simulink library "EngineSystemSubmodel"  (R2014b)
settings: Solver=ode45  StartTime=0.0  StopTime=10.0  FixedStep=1e-4  RelTol=1e-3
values from neighbouring files (symbols this model uses):
  D_turb_wheel = TC.TC_map.turb.D_wheel    [init_MVM.m]
  delta = 2    [Init8RTFLEX68D.m]    (also in Untitled2.m = fcn(p); fcn.m = zeros(size(p)))
  eta_turb_max = TC.TC_map.turb.eff_max    [init_MVM.m]
  flow_coeff_turb = [-1.585326540339;-4.823836967181;1.5853156139822]    [Init8RTFLEX68D.m]    (also in init_MVM.m = TC.TC_map.turb.flow_fit_coeff)
  fs = 0.0683    [Init8RTFLEX68D.m]    (also in NOxProcessGUI.m = varargin{2}; initHybrid.m; initMV.m; init_MVM.m = 0.0682925799315)
  genset = generators(1)    [runTempCyl4S.m]
  J_tc = TC.SAE_map_comp.inertia    [init_MVM.m]
  kai = 1.7    [Init8RTFLEX68D.m]
  Kb = 1*ones(engines,1)    [initHybrid.m]    (also in initMV.m; init_MVM.m = 1; init_ele.m = 1)
  Kd = 20*ones(engines,1)    [initHybrid.m]    (also in initMV.m; init_MVM.m = 10; init_ele.m = 20)
  Ki = 20*ones(engines,1)    [initHybrid.m]    (also in initMV.m; init_MVM.m = 10; init_ele.m = 20)
  Kp = 20*ones(engines,1)    [initHybrid.m]    (also in initMV.m; init_MVM.m = 10; init_ele.m = 20)
  Load_amp = x(4) + xRef(i)    [GetErrGensetResp.m]    (also in runsimulation.m = 0.55; runsimulationRecovery.m = InitialLoad(jj) + LoadStep(ii))
  Load_bias = x(4)    [GetErrGensetResp.m]    (also in runsimulation.m = 0.15; runsimulationRecovery.m = InitialLoad(jj))
  Load_index = 1    [GetErrGensetResp.m]    (also in runsimulation.m; runsimulationRecovery.m)
  N = x*noMol    [NOxProcessGUI.m]    (also in initHybrid.m = .1*ones(engines,1); initMV.m = .1*ones(engines,1); init_ele.m = 0.1)
  omegat0 = RPM_TC_initial/30*pi    [init_MVM.m]
  Start_time = 50    [GetErrGensetResp.m]    (also in runsimulation.m; runsimulationRecovery.m)
  T_load = 1    [GetErrGensetResp.m]    (also in runsimulation.m; runsimulationRecovery.m)
  T_ref_turb = TC.TC_map.turb.T_ref    [init_MVM.m]
  u0 = 0.2    [init_MVM.m]
  Uc_opt = TC.TC_map.turb.Uc_opt    [init_MVM.m]
  uMax = 1.5*ones(engines,1)    [initHybrid.m]    (also in initMV.m; init_MVM.m = 1.1; init_ele.m = 1.1)
  uMin = 0*ones(engines,1)    [initHybrid.m]    (also in initMV.m; init_MVM.m = 0.1; init_ele.m = 0.1)
undefined symbols (not defined in the file or in its folder): CAIPO, control, CV, cyl, eng, engSCont, omega0, rhoG0, Td, Ti, turbo, u_max, volDisp, vSCont, vSDes
undefined symbols (not defined in the file): comp_eff_map, comp_flow_map, n288_rep, npr, nsp, pr_rep, vComp
libraries: EngineSystemSubmodel x167, simulink x2
(part 2 of 5)

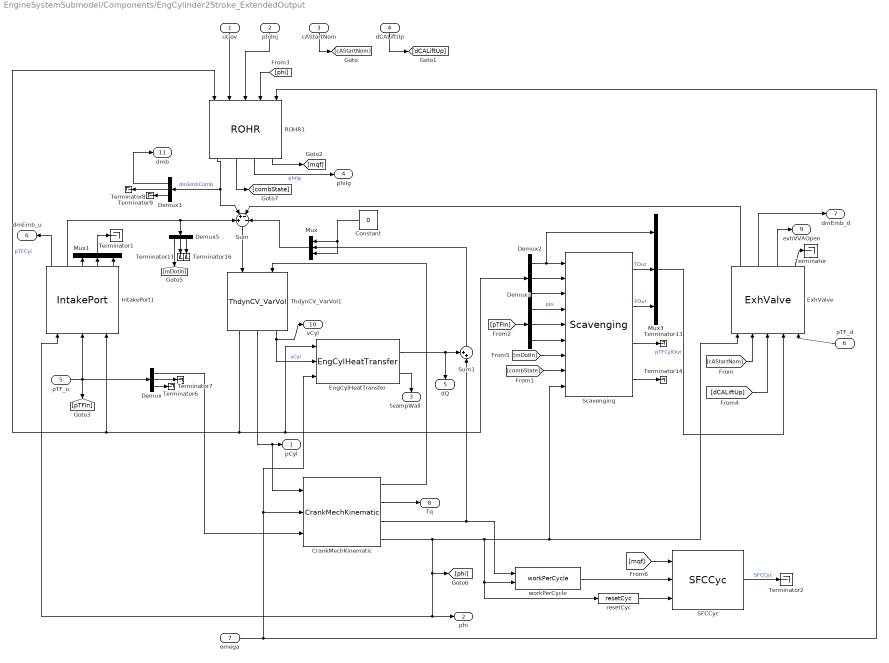
== system EngineSystemSubmodel/Components/EngCylinder2Stroke_ExtendedOutput ==
  uGov : Inport
  phiInj : Inport  Port=2
  cAStartNom : Inport  Port=3
  dCALiftUp : Inport  Port=4
  pTF_u : Inport  Port=5
  pTF_d : Inport  Port=6
  omega : Inport  Port=7
  Constant : Constant  Value=0
  CrankMechKinematic : EngineSystemSubmodel/Mechanical Part/CrankMechKinematic
  Demux{,1..3,5} (5 alike) : Demux  Outputs=3
  EngCylHeatTransfer : EngineSystemSubmodel/Heat Transfer/EngCylHeatTransfer
  ExhValve : EngineSystemSubmodel/Components/ExhValve
  IntakePort1 : EngineSystemSubmodel/Components/IntakePort
  Mux : Mux  Inputs=3
  Mux1 : Mux  Inputs=3
  Mux3 : Mux  Inputs=3
  ROHR1 : EngineSystemSubmodel/Combustion/ROHR
  SFCCyc : EngineSystemSubmodel/EngineOperatingParameterCalculation/SFCCyc
  Scavenging : EngineSystemSubmodel/Gas Exchange/Scavenging
  Sum : Sum  Inputs=++--
  Sum1 : Sum  Inputs=++|
  Terminator{,1..2,6..9,11,13..14,16} (11 alike) : Terminator
  ThdynCV_VarVol1 : EngineSystemSubmodel/Control Volume/ThdynCV_VarVol  CV=cyl.init
  resetCyc : EngineSystemSubmodel/EngineOperatingParameterCalculation/resetCyc
  workPerCycle : EngineSystemSubmodel/EngineOperatingParameterCalculation/workPerCycle
  pCyl : Outport
  phi : Outport  Port=2
  teampWall : Outport  Port=3
  phiIg : Outport  Port=4
  dQ : Outport  Port=5
  dmEmb_u : Outport  Port=6
  dmEmb_d : Outport  Port=7
  Tq : Outport  Port=8
  exhVVAOpen : Outport  Port=9
  vCyl : Outport  Port=10
  dmb : Outport  Port=11
  wires:
  SFCCyc/1 -> Terminator2/1  "SFCCyc"
  [mqf] -> SFCCyc/1
  workPerCycle/1 -> SFCCyc/2
  resetCyc/1 -> SFCCyc/3
  Mux3/1 -> ExhValve/4  "pTFCylOut"
  [cAStartNom] -> ExhValve/2
  dCALiftUp/1 -> [dCALiftUp]
  cAStartNom/1 -> [cAStartNom]
  ExhValve/2 -> dmEmb_d/1
  ExhValve/4 -> Terminator/1
  ExhValve/3 -> exhVVAOpen/1
  Mux1/1 -> Terminator1/1
  IntakePort1/5 -> Mux1/3
  IntakePort1/4 -> Mux1/2
  IntakePort1/3 -> Mux1/1
  ROHR1/3 -> phiIg/1  "phiIg"
  EngCylHeatTransfer/2 -> teampWall/1
  Demux/3 -> Terminator7/1
  Demux/2 -> Terminator6/1
  Constant/1 -> Mux/3, Mux/1
  Mux/1 -> Sum/4
  Sum1/1 -> Mux/2
  EngCylHeatTransfer/1 -> Sum1/1, dQ/1
  ThdynCV_VarVol1/3 -> EngCylHeatTransfer/2, vCyl/1  "vCyl"
  IntakePort1/1 -> dmEmb_u/1
  omega/1 -> ROHR1/5, EngCylHeatTransfer/3, CrankMechKinematic/2
  phiInj/1 -> ROHR1/3
  CrankMechKinematic/2 -> Tq/1
  Demux/1 -> CrankMechKinematic/3
  CrankMechKinematic/3 -> Sum1/2, workPerCycle/1
  uGov/1 -> ROHR1/2
  CrankMechKinematic/1 -> ThdynCV_VarVol1/2
  ThdynCV_VarVol1/2 -> CrankMechKinematic/1, pCyl/1
  ThdynCV_VarVol1/1 -> EngCylHeatTransfer/1, Demux2/1, IntakePort1/3, ROHR1/1  "pTFCyl"
  Sum/1 -> ThdynCV_VarVol1/1
  ExhValve/1 -> Sum/3
  ROHR1/1 -> Sum/2, Demux1/1  "dmEmbComb"
  Demux1/1 -> dmb/1
  Demux1/2 -> Terminator8/1
  Demux1/3 -> Terminator9/1
  ROHR1/4 -> [mqf]
  pTF_u/1 -> [pTFIn], Demux/1, IntakePort1/2
  pTF_d/1 -> ExhValve/5
  ROHR1/2 -> [combState]
  [pTFIn] -> Demux3/1
  Demux3/1 -> Scavenging/4  "pIn"
  Demux3/2 -> Scavenging/5
  Demux3/3 -> Scavenging/6
  [mDotIn] -> Scavenging/7
  CrankMechKinematic/4 -> [phi], IntakePort1/1, phi/1, Scavenging/9, ExhValve/1, workPerCycle/2, resetCyc/1
  IntakePort1/2 -> Demux5/1, Sum/1
  Demux5/2 -> Terminator11/1
  Demux5/3 -> Terminator16/1
  Demux5/1 -> [mDotIn]
  [combState] -> Scavenging/8
  [phi] -> ROHR1/4
  Scavenging/3 -> Terminator13/1
  Scavenging/4 -> Terminator14/1
  Demux2/2 -> Scavenging/2
  Demux2/1 -> Mux3/1, Scavenging/1
  Demux2/3 -> Scavenging/3
  Scavenging/1 -> Mux3/2  "TOut"
  Scavenging/2 -> Mux3/3  "FOut"
  [dCALiftUp] -> ExhValve/3

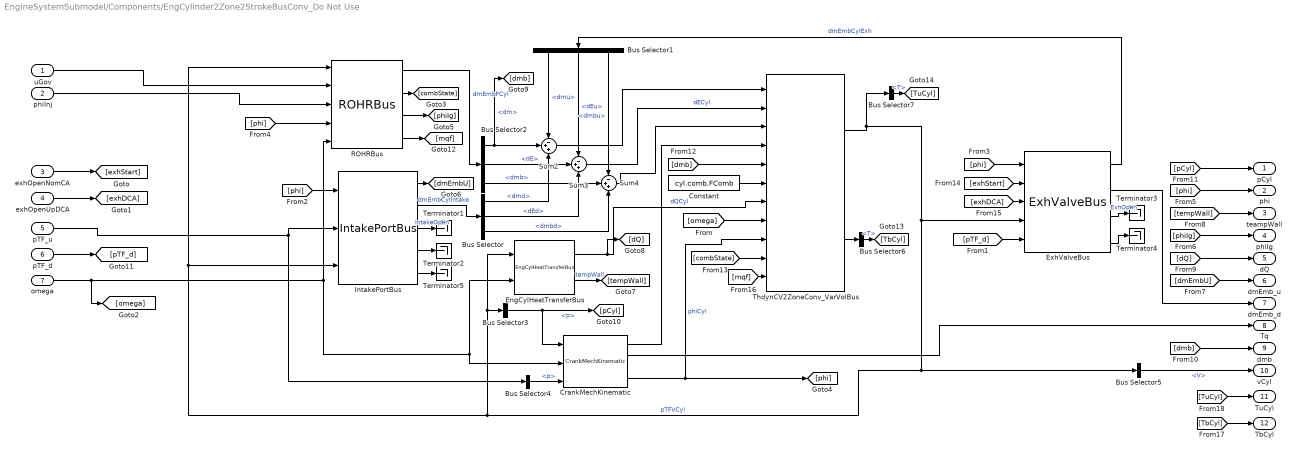
== system EngineSystemSubmodel/Components/EngCylinder2Zone2StrokeBusConv_Do Not Use ==
  uGov : Inport
  phiInj : Inport  Port=2
  exhOpenNomCA : Inport  Port=3
  exhOpenUpDCA : Inport  Port=4
  pTF_u : Inport  Port=5
  pTF_d : Inport  Port=6
  omega : Inport  Port=7
  Bus Selector : BusSelector  OutputSignals=dmd,dEd,dmbd
  Bus Selector1 : BusSelector  OutputSignals=dmu,dEu,dmbu
  Bus Selector2 : BusSelector  OutputSignals=dm,dE,dmb
  Bus Selector3 : BusSelector  OutputSignals=p
  Bus Selector4 : BusSelector  OutputSignals=p
  Bus Selector5 : BusSelector  OutputSignals=V
  Bus Selector6 : BusSelector  OutputSignals=T
  Bus Selector7 : BusSelector  OutputSignals=T
  Constant : Constant  Value=cyl.comb.FComb
  CrankMechKinematic : EngineSystemSubmodel/Mechanical Part/CrankMechKinematic
  EngCylHeatTransferBus : EngineSystemSubmodel/Heat Transfer/EngCylHeatTransferBus
  ExhValveBus : EngineSystemSubmodel/Components/ExhValveBus
  IntakePortBus : EngineSystemSubmodel/Components/IntakePortBus
  ROHRBus : EngineSystemSubmodel/Combustion/ROHRBus
  Sum2 : Sum  Inputs=-++
  Sum3 : Sum  Inputs=-++
  Sum4 : Sum  Inputs=-++
  Terminator{1..5} (5 alike) : Terminator
  ThdynCV2ZoneConv_VarVolBus : EngineSystemSubmodel/Control Volume/ThdynCV2ZoneConv_VarVolBus  CV=cyl.init
  pCyl : Outport
  phi : Outport  Port=2
  teampWall : Outport  Port=3
  phiIg : Outport  Port=4
  dQ : Outport  Port=5
  dmEmb_u : Outport  Port=6
  dmEmb_d : Outport  Port=7
  Tq : Outport  Port=8
  dmb : Outport  Port=9
  vCyl : Outport  Port=10
  TuCyl : Outport  Port=11
  TbCyl : Outport  Port=12
  wires:
  ROHRBus/4 -> [mqf]
  Bus Selector5/1 -> vCyl/1  "<V>"
  IntakePortBus/5 -> Terminator5/1
  [pTF_d] -> ExhValveBus/5
  pTF_d/1 -> [pTF_d]
  phiInj/1 -> ROHRBus/3
  uGov/1 -> ROHRBus/2
  Bus Selector2/2 -> Sum3/2  "<dE>"
  ExhValveBus/4 -> Terminator4/1
  ExhValveBus/3 -> Terminator3/1  "ExhOpen"
  IntakePortBus/4 -> Terminator2/1
  IntakePortBus/3 -> Terminator1/1  "IntakeOpen"
  ROHRBus/2 -> [combState]
  [exhDCA] -> ExhValveBus/3
  [exhStart] -> ExhValveBus/2
  [pCyl] -> pCyl/1
  [dmb] -> dmb/1
  [dQ] -> dQ/1
  [tempWall] -> teampWall/1
  EngCylHeatTransferBus/2 -> [tempWall]  "tempWall"
  ExhValveBus/2 -> dmEmb_d/1
  [dmEmbU] -> dmEmb_u/1
  IntakePortBus/1 -> [dmEmbU]
  [phi] -> phi/1
  [phiIg] -> phiIg/1
  ROHRBus/3 -> [phiIg]
  [phi] -> ROHRBus/4
  exhOpenUpDCA/1 -> [exhDCA]
  exhOpenNomCA/1 -> [exhStart]
  Bus Selector4/1 -> CrankMechKinematic/3  "<p>"
  pTF_u/1 -> Bus Selector4/1, IntakePortBus/2
  [phi] -> ExhValveBus/1
  [phi] -> IntakePortBus/1
  CrankMechKinematic/4 -> ThdynCV2ZoneConv_VarVolBus/9, [phi]  "phiCyl"
  EngCylHeatTransferBus/1 -> ThdynCV2ZoneConv_VarVolBus/7, [dQ]  "dQCyl"
  CrankMechKinematic/1 -> ThdynCV2ZoneConv_VarVolBus/4
  CrankMechKinematic/2 -> Tq/1
  Bus Selector3/1 -> [pCyl], CrankMechKinematic/1  "<p>"
  omega/1 -> [omega], EngCylHeatTransferBus/2, CrankMechKinematic/2, ROHRBus/5
  Bus Selector2/3 -> Sum4/2  "<dmb>"
  Bus Selector/3 -> Sum4/3  "<dmbd>"
  Bus Selector/2 -> Sum3/3  "<dEd>"
  Bus Selector2/1 -> Sum2/2, [dmb]  "<dm>"
  ROHRBus/1 -> Bus Selector2/1  "dmEmbFCyl"
  Bus Selector/1 -> Sum2/3  "<dmd>"
  ThdynCV2ZoneConv_VarVolBus/1 -> Bus Selector7/1, ExhValveBus/4, Bus Selector3/1, EngCylHeatTransferBus/1, IntakePortBus/3, ROHRBus/1, Bus Selector5/1  "pTFVCyl"
  Bus Selector1/3 -> Sum4/1  "<dmbu>"
  Bus Selector1/2 -> Sum3/1  "<dEu>"
  Bus Selector1/1 -> Sum2/1  "<dmu>"
  ExhValveBus/1 -> Bus Selector1/1  "dmEmbCylExh"
  Sum4/1 -> ThdynCV2ZoneConv_VarVolBus/3
  Sum3/1 -> ThdynCV2ZoneConv_VarVolBus/2  "dECyl"
  Sum2/1 -> ThdynCV2ZoneConv_VarVolBus/1
  IntakePortBus/2 -> Bus Selector/1  "dmEmbCylIntake"
  [dmb] -> ThdynCV2ZoneConv_VarVolBus/5
  Constant/1 -> ThdynCV2ZoneConv_VarVolBus/6
  [omega] -> ThdynCV2ZoneConv_VarVolBus/8
  [combState] -> ThdynCV2ZoneConv_VarVolBus/10
  [mqf] -> ThdynCV2ZoneConv_VarVolBus/11
  ThdynCV2ZoneConv_VarVolBus/2 -> Bus Selector6/1
  Bus Selector6/1 -> [TbCyl]  "<T>"
  [TbCyl] -> TbCyl/1
  Bus Selector7/1 -> [TuCyl]  "<T>"
  [TuCyl] -> TuCyl/1

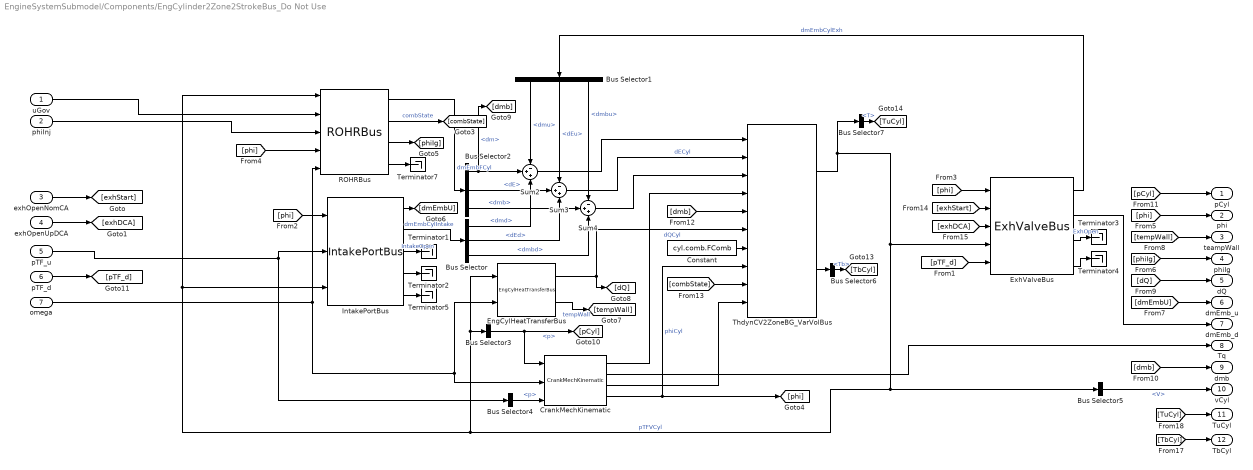
== system EngineSystemSubmodel/Components/EngCylinder2Zone2StrokeBus_Do Not Use ==
  uGov : Inport
  phiInj : Inport  Port=2
  exhOpenNomCA : Inport  Port=3
  exhOpenUpDCA : Inport  Port=4
  pTF_u : Inport  Port=5
  pTF_d : Inport  Port=6
  omega : Inport  Port=7
  Bus Selector : BusSelector  OutputSignals=dmd,dEd,dmbd
  Bus Selector1 : BusSelector  OutputSignals=dmu,dEu,dmbu
  Bus Selector2 : BusSelector  OutputSignals=dm,dE,dmb
  Bus Selector3 : BusSelector  OutputSignals=p
  Bus Selector4 : BusSelector  OutputSignals=p
  Bus Selector5 : BusSelector  OutputSignals=V
  Bus Selector6 : BusSelector  OutputSignals=Tb
  Bus Selector7 : BusSelector  OutputSignals=T
  Constant : Constant  Value=cyl.comb.FComb
  CrankMechKinematic : EngineSystemSubmodel/Mechanical Part/CrankMechKinematic
  EngCylHeatTransferBus : EngineSystemSubmodel/Heat Transfer/EngCylHeatTransferBus
  ExhValveBus : EngineSystemSubmodel/Components/ExhValveBus
  IntakePortBus : EngineSystemSubmodel/Components/IntakePortBus
  ROHRBus : EngineSystemSubmodel/Combustion/ROHRBus
  Sum2 : Sum  Inputs=-++
  Sum3 : Sum  Inputs=-++
  Sum4 : Sum  Inputs=-++
  Terminator{1..5,7} (6 alike) : Terminator
  ThdynCV2ZoneBG_VarVolBus : EngineSystemSubmodel/Control Volume/ThdynCV2ZoneBG_VarVolBus  CV=cyl.init
  pCyl : Outport
  phi : Outport  Port=2
  teampWall : Outport  Port=3
  phiIg : Outport  Port=4
  dQ : Outport  Port=5
  dmEmb_u : Outport  Port=6
  dmEmb_d : Outport  Port=7
  Tq : Outport  Port=8
  dmb : Outport  Port=9
  vCyl : Outport  Port=10
  TuCyl : Outport  Port=11
  TbCyl : Outport  Port=12
  wires:
  ROHRBus/2 -> [combState]  "combState"
  CrankMechKinematic/3 -> ThdynCV2ZoneBG_VarVolBus/10
  ROHRBus/4 -> Terminator7/1
  Bus Selector5/1 -> vCyl/1  "<V>"
  IntakePortBus/5 -> Terminator5/1
  [pTF_d] -> ExhValveBus/5
  pTF_d/1 -> [pTF_d]
  phiInj/1 -> ROHRBus/3
  uGov/1 -> ROHRBus/2
  Bus Selector2/2 -> Sum3/2  "<dE>"
  ExhValveBus/4 -> Terminator4/1
  ExhValveBus/3 -> Terminator3/1  "ExhOpen"
  IntakePortBus/4 -> Terminator2/1
  IntakePortBus/3 -> Terminator1/1  "IntakeOpen"
  [exhDCA] -> ExhValveBus/3
  [exhStart] -> ExhValveBus/2
  [pCyl] -> pCyl/1
  [dmb] -> dmb/1
  [dQ] -> dQ/1
  [tempWall] -> teampWall/1
  EngCylHeatTransferBus/2 -> [tempWall]  "tempWall"
  ExhValveBus/2 -> dmEmb_d/1
  [dmEmbU] -> dmEmb_u/1
  IntakePortBus/1 -> [dmEmbU]
  [phi] -> phi/1
  [phiIg] -> phiIg/1
  ROHRBus/3 -> [phiIg]
  [phi] -> ROHRBus/4
  exhOpenUpDCA/1 -> [exhDCA]
  exhOpenNomCA/1 -> [exhStart]
  Bus Selector4/1 -> CrankMechKinematic/3  "<p>"
  pTF_u/1 -> Bus Selector4/1, IntakePortBus/2
  [phi] -> ExhValveBus/1
  [phi] -> IntakePortBus/1
  CrankMechKinematic/4 -> ThdynCV2ZoneBG_VarVolBus/8, [phi]  "phiCyl"
  EngCylHeatTransferBus/1 -> [dQ], ThdynCV2ZoneBG_VarVolBus/6  "dQCyl"
  CrankMechKinematic/1 -> ThdynCV2ZoneBG_VarVolBus/4
  CrankMechKinematic/2 -> Tq/1
  Bus Selector3/1 -> [pCyl], CrankMechKinematic/1  "<p>"
  omega/1 -> EngCylHeatTransferBus/2, CrankMechKinematic/2, ROHRBus/5
  Bus Selector2/3 -> Sum4/2  "<dmb>"
  Bus Selector/3 -> Sum4/3  "<dmbd>"
  Bus Selector/2 -> Sum3/3  "<dEd>"
  Bus Selector2/1 -> Sum2/2, [dmb]  "<dm>"
  ROHRBus/1 -> Bus Selector2/1  "dmEmbFCyl"
  Bus Selector/1 -> Sum2/3  "<dmd>"
  ThdynCV2ZoneBG_VarVolBus/1 -> Bus Selector7/1, ExhValveBus/4, Bus Selector3/1, EngCylHeatTransferBus/1, IntakePortBus/3, ROHRBus/1, Bus Selector5/1  "pTFVCyl"
  Bus Selector1/3 -> Sum4/1  "<dmbu>"
  Bus Selector1/2 -> Sum3/1  "<dEu>"
  Bus Selector1/1 -> Sum2/1  "<dmu>"
  ExhValveBus/1 -> Bus Selector1/1  "dmEmbCylExh"
  Sum4/1 -> ThdynCV2ZoneBG_VarVolBus/3
  Sum3/1 -> ThdynCV2ZoneBG_VarVolBus/2  "dECyl"
  Sum2/1 -> ThdynCV2ZoneBG_VarVolBus/1
  IntakePortBus/2 -> Bus Selector/1  "dmEmbCylIntake"
  [dmb] -> ThdynCV2ZoneBG_VarVolBus/5
  Constant/1 -> ThdynCV2ZoneBG_VarVolBus/7
  [combState] -> ThdynCV2ZoneBG_VarVolBus/9
  ThdynCV2ZoneBG_VarVolBus/2 -> Bus Selector6/1
  Bus Selector6/1 -> [TbCyl]  "<Tb>"
  [TbCyl] -> TbCyl/1
  Bus Selector7/1 -> [TuCyl]  "<T>"
  [TuCyl] -> TuCyl/1

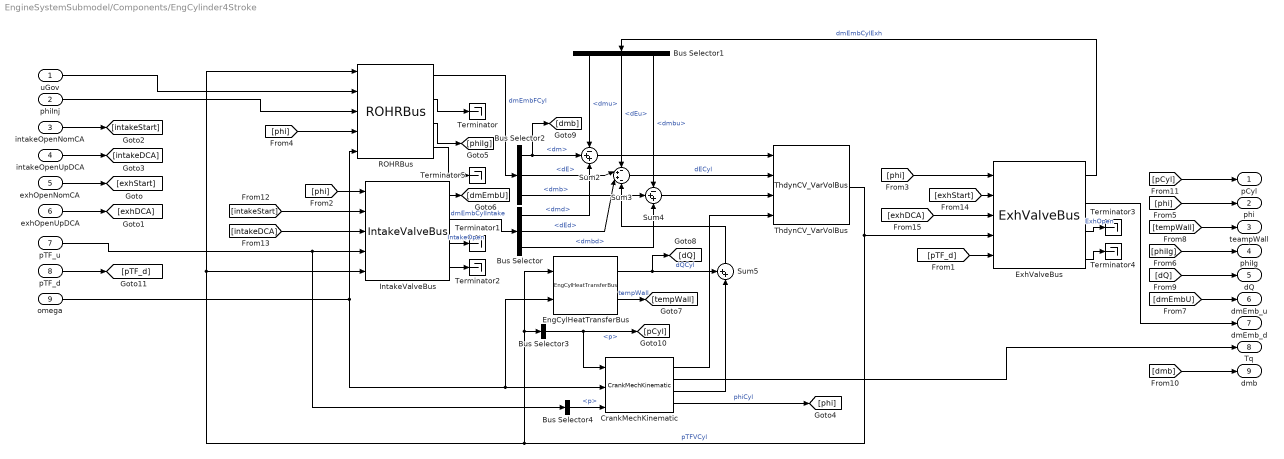
== system EngineSystemSubmodel/Components/EngCylinder4Stroke ==
  uGov : Inport
  phiInj : Inport  Port=2
  intakeOpenNomCA : Inport  Port=3
  intakeOpenUpDCA : Inport  Port=4
  exhOpenNomCA : Inport  Port=5
  exhOpenUpDCA : Inport  Port=6
  pTF_u : Inport  Port=7
  pTF_d : Inport  Port=8
  omega : Inport  Port=9
  Bus Selector : BusSelector  OutputSignals=dmd,dEd,dmbd
  Bus Selector1 : BusSelector  OutputSignals=dmu,dEu,dmbu
  Bus Selector2 : BusSelector  OutputSignals=dm,dE,dmb
  Bus Selector3 : BusSelector  OutputSignals=p
  Bus Selector4 : BusSelector  OutputSignals=p
  CrankMechKinematic : EngineSystemSubmodel/Mechanical Part/CrankMechKinematic
  EngCylHeatTransferBus : EngineSystemSubmodel/Heat Transfer/EngCylHeatTransferBus
  ExhValveBus : EngineSystemSubmodel/Components/ExhValveBus
  IntakeValveBus : EngineSystemSubmodel/Components/IntakeValveBus
  ROHRBus : EngineSystemSubmodel/Combustion/ROHRBus
  Sum2 : Sum  Inputs=-++
  Sum3 : Sum  Inputs=-++-
  Sum4 : Sum  Inputs=-++
  Sum5 : Sum  Inputs=++|
  Terminator{,1..5} (6 alike) : Terminator
  ThdynCV_VarVolBus : EngineSystemSubmodel/Control Volume/ThdynCV_VarVolBus  CV=cyl.init
  pCyl : Outport
  phi : Outport  Port=2
  teampWall : Outport  Port=3
  phiIg : Outport  Port=4
  dQ : Outport  Port=5
  dmEmb_u : Outport  Port=6
  dmEmb_d : Outport  Port=7
  Tq : Outport  Port=8
  dmb : Outport  Port=9
  wires:
  IntakeValveBus/2 -> Bus Selector/1  "dmEmbCylIntake"
  Sum2/1 -> ThdynCV_VarVolBus/1
  Sum3/1 -> ThdynCV_VarVolBus/2  "dECyl"
  Sum4/1 -> ThdynCV_VarVolBus/3
  ExhValveBus/1 -> Bus Selector1/1  "dmEmbCylExh"
  Bus Selector1/1 -> Sum2/1  "<dmu>"
  Bus Selector1/2 -> Sum3/1  "<dEu>"
  Bus Selector1/3 -> Sum4/1  "<dmbu>"
  ThdynCV_VarVolBus/1 -> ExhValveBus/4, ROHRBus/1, IntakeValveBus/5, EngCylHeatTransferBus/1, Bus Selector3/1  "pTFVCyl"
  Bus Selector/1 -> Sum2/3  "<dmd>"
  ROHRBus/1 -> Bus Selector2/1  "dmEmbFCyl"
  Bus Selector2/1 -> [dmb], Sum2/2  "<dm>"
  Bus Selector/2 -> Sum3/3  "<dEd>"
  Bus Selector/3 -> Sum4/3  "<dmbd>"
  Bus Selector2/3 -> Sum4/2  "<dmb>"
  omega/1 -> ROHRBus/5, EngCylHeatTransferBus/2, CrankMechKinematic/2
  Bus Selector3/1 -> CrankMechKinematic/1, [pCyl]  "<p>"
  CrankMechKinematic/2 -> Tq/1
  CrankMechKinematic/1 -> ThdynCV_VarVolBus/4
  EngCylHeatTransferBus/1 -> [dQ], Sum5/1  "dQCyl"
  CrankMechKinematic/4 -> [phi]  "phiCyl"
  [phi] -> IntakeValveBus/1
  [phi] -> ExhValveBus/1
  pTF_u/1 -> Bus Selector4/1, IntakeValveBus/4
  Bus Selector4/1 -> CrankMechKinematic/3  "<p>"
  intakeOpenNomCA/1 -> [intakeStart]
  intakeOpenUpDCA/1 -> [intakeDCA]
  exhOpenNomCA/1 -> [exhStart]
  exhOpenUpDCA/1 -> [exhDCA]
  [phi] -> ROHRBus/4
  ROHRBus/3 -> [phiIg]
  [phiIg] -> phiIg/1
  [phi] -> phi/1
  IntakeValveBus/1 -> [dmEmbU]
  [dmEmbU] -> dmEmb_u/1
  ExhValveBus/2 -> dmEmb_d/1
  EngCylHeatTransferBus/2 -> [tempWall]  "tempWall"
  [tempWall] -> teampWall/1
  [dQ] -> dQ/1
  [dmb] -> dmb/1
  [pCyl] -> pCyl/1
  [intakeStart] -> IntakeValveBus/2
  [intakeDCA] -> IntakeValveBus/3
  [exhStart] -> ExhValveBus/2
  [exhDCA] -> ExhValveBus/3
  ROHRBus/2 -> Terminator/1
  IntakeValveBus/3 -> Terminator1/1  "IntakeOpen"
  IntakeValveBus/4 -> Terminator2/1
  ExhValveBus/3 -> Terminator3/1  "ExhOpen"
  ExhValveBus/4 -> Terminator4/1
  Sum5/1 -> Sum3/4
  Bus Selector2/2 -> Sum3/2  "<dE>"
  uGov/1 -> ROHRBus/2
  phiInj/1 -> ROHRBus/3
  pTF_d/1 -> [pTF_d]
  [pTF_d] -> ExhValveBus/5
  CrankMechKinematic/3 -> Sum5/2
  ROHRBus/4 -> Terminator5/1

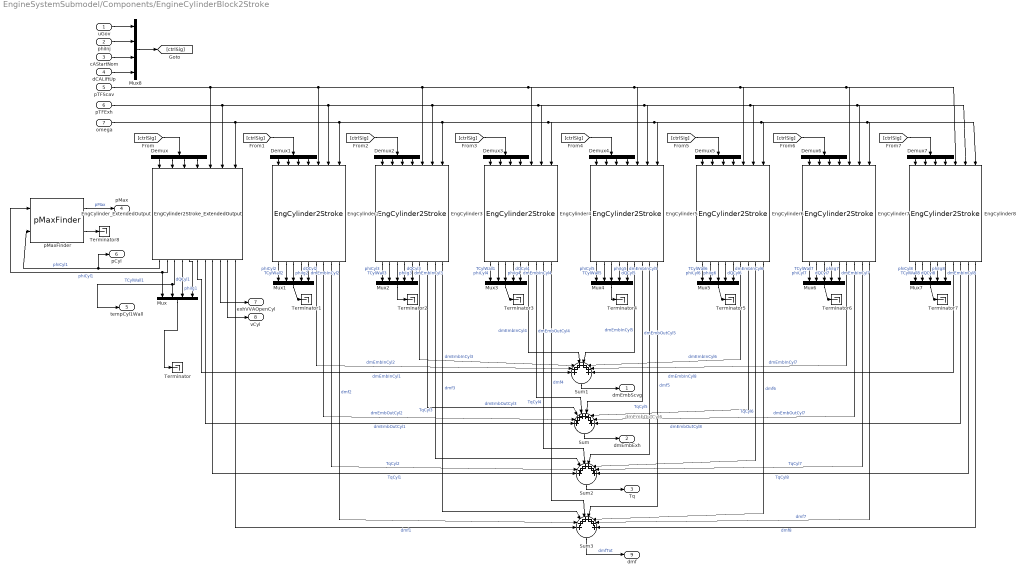
== system EngineSystemSubmodel/Components/EngineCylinderBlock2Stroke ==
  note: dmEmbOutCyl6
  uGov : Inport
  phiInj : Inport  Port=2
  cAStartNom : Inport  Port=3
  dCALiftUp : Inport  Port=4
  pTFScav : Inport  Port=5
  pTFExh : Inport  Port=6
  omega : Inport  Port=7
  Demux{,1..7} (8 alike) : Demux
  EngCylinder2 : EngineSystemSubmodel/Components/EngCylinder2Stroke  cylPar=eng.cyl  cylNo=2  cyl=eng.cyl
  EngCylinder3 : EngineSystemSubmodel/Components/EngCylinder2Stroke  cylPar=eng.cyl  cylNo=3  cyl=eng.cyl
  EngCylinder4 : EngineSystemSubmodel/Components/EngCylinder2Stroke  cylPar=eng.cyl  cylNo=4  cyl=eng.cyl
  EngCylinder5 : EngineSystemSubmodel/Components/EngCylinder2Stroke  cylPar=eng.cyl  cylNo=5  cyl=eng.cyl
  EngCylinder6 : EngineSystemSubmodel/Components/EngCylinder2Stroke  cylPar=eng.cyl  cylNo=6  cyl=eng.cyl
  EngCylinder7 : EngineSystemSubmodel/Components/EngCylinder2Stroke  cylPar=eng.cyl  cylNo=7  cyl=eng.cyl
  EngCylinder8 : EngineSystemSubmodel/Components/EngCylinder2Stroke  cylPar=eng.cyl  cylNo=8  cyl=eng.cyl
  EngCylinder_ExtendedOutput : EngineSystemSubmodel/Components/EngCylinder2Stroke_ExtendedOutput  cylPar=eng.cyl  cylNo=1  cyl=eng.cyl
  Mux : Mux
  Mux{1..7} (7 alike) : Mux  Inputs=5
  Mux8 : Mux
  Sum{,1..3} (4 alike) : Sum  Inputs=++++++++
  Terminator{,1..8} (9 alike) : Terminator
  pMaxFinder : EngineSystemSubmodel/EngineOperatingParameterCalculation/pMaxFinder
  dmEmbScvg : Outport
  dmEmbExh : Outport  Port=2
  Tq : Outport  Port=3
  pMax : Outport  Port=4
  tempCyl1Wall : Outport  Port=5
  pCyl : Outport  Port=6
  exhVVAOpenCyl : Outport  Port=7
  vCyl : Outport  Port=8
  dmf : Outport  Port=9
  wires:
  EngCylinder8/7 -> Sum/8  "dmEmbOutCyl8"
  EngCylinder7/7 -> Sum/7  "dmEmbOutCyl7"
  EngCylinder8/5 -> Mux7/5  "dmEmbInCyl8"
  EngCylinder8/4 -> Mux7/4  "dQCyl8"
  EngCylinder7/5 -> Mux6/5  "dmEmbInCyl7"
  EngCylinder2/8 -> Sum2/2  "TqCyl2"
  EngCylinder7/8 -> Sum2/7  "TqCyl7"
  EngCylinder8/8 -> Sum2/8  "TqCyl8"
  EngCylinder6/8 -> Sum2/6  "TqCyl6"
  pTFScav/1 -> EngCylinder_ExtendedOutput/5, EngCylinder2/5, EngCylinder4/5, EngCylinder5/5, EngCylinder8/5, EngCylinder7/5, EngCylinder6/5, EngCylinder3/5
  EngCylinder3/8 -> Sum2/3  "TqCyl3"
  EngCylinder4/8 -> Sum2/4  "TqCyl4"
  EngCylinder5/8 -> Sum2/5  "TqCyl5"
  EngCylinder_ExtendedOutput/6 -> Sum1/1  "dmEmbInCyl1"
  EngCylinder2/6 -> Sum1/2  "dmEmbInCyl2"
  EngCylinder3/6 -> Sum1/3  "dmEmbInCyl3"
  EngCylinder4/6 -> Sum1/4  "dmEmbInCyl4"
  EngCylinder6/6 -> Sum1/6  "dmEmbInCyl6"
  EngCylinder5/6 -> Sum1/5  "dmEmbInCyl5"
  EngCylinder4/7 -> Sum/4  "dmEmbOutCyl4"
  EngCylinder3/7 -> Sum/3  "dmEmbOutCyl3"
  EngCylinder_ExtendedOutput/7 -> Sum/1  "dmEmbOutCyl1"
  EngCylinder7/6 -> Sum1/7  "dmEmbInCyl7"
  EngCylinder2/7 -> Sum/2  "dmEmbOutCyl2"
  EngCylinder6/7 -> Sum/6
  EngCylinder5/7 -> Sum/5  "dmEmbOutCyl5"
  Mux7/1 -> Terminator7/1
  EngCylinder8/3 -> Mux7/3  "phiIg8"
  EngCylinder8/2 -> Mux7/2  "TCylWall8"
  EngCylinder8/1 -> Mux7/1  "phiCyl8"
  EngCylinder4/3 -> Mux3/3  "phiIg4"
  EngCylinder3/2 -> Mux2/2  "TCylWall3"
  Mux2/1 -> Terminator2/1
  EngCylinder5/2 -> Mux4/2  "TCylWall5"
  EngCylinder4/4 -> Mux3/4  "dQCyl4"
  EngCylinder4/1 -> Mux3/1  "phiCyl4"
  EngCylinder5/1 -> Mux4/1  "phiCyl5"
  Mux/1 -> Terminator/1
  Mux3/1 -> Terminator3/1
  EngCylinder3/1 -> Mux2/1  "phiCyl3"
  EngCylinder2/2 -> Mux1/2  "TCylWall2"
  EngCylinder2/3 -> Mux1/3  "phiIg2"
  EngCylinder4/2 -> Mux3/2  "TCylWall1"
  EngCylinder3/3 -> Mux2/3  "phiIg3"
  EngCylinder_ExtendedOutput/2 -> pMaxFinder/1, Mux/1  "phiCyl1"
  EngCylinder3/4 -> Mux2/4  "dQCyl3"
  Mux4/1 -> Terminator4/1
  EngCylinder2/4 -> Mux1/4  "dQCyl2"
  EngCylinder5/4 -> Mux4/4  "dQCyl5"
  EngCylinder_ExtendedOutput/5 -> Mux/4  "dQCyl1"
  EngCylinder_ExtendedOutput/4 -> Mux/3  "phiIg1"
  EngCylinder5/3 -> Mux4/3  "phiIg5"
  Mux1/1 -> Terminator1/1
  EngCylinder2/1 -> Mux1/1  "phiCyl2"
  EngCylinder_ExtendedOutput/3 -> tempCyl1Wall/1, Mux/2  "TCylWall1"
  EngCylinder6/4 -> Mux5/4  "dQCyl6"
  Mux5/1 -> Terminator5/1
  EngCylinder6/3 -> Mux5/3  "phiIg6"
  pTFExh/1 -> EngCylinder_ExtendedOutput/6, EngCylinder8/6, EngCylinder7/6, EngCylinder6/6, EngCylinder5/6, EngCylinder4/6, EngCylinder3/6, EngCylinder2/6
  EngCylinder6/1 -> Mux5/1  "phiCyl6"
  EngCylinder6/2 -> Mux5/2  "TCylWall6"
  omega/1 -> EngCylinder_ExtendedOutput/7, EngCylinder3/7, EngCylinder4/7, EngCylinder5/7, EngCylinder6/7, EngCylinder7/7, EngCylinder8/7, EngCylinder2/7
  EngCylinder7/1 -> Mux6/1  "phiCyl7"
  EngCylinder_ExtendedOutput/8 -> Sum2/1  "TqCyl1"
  EngCylinder7/4 -> Mux6/4  "dQCyl7"
  EngCylinder7/2 -> Mux6/2  "TCylWall7"
  EngCylinder8/6 -> Sum1/8  "dmEmbInCyl8"
  EngCylinder7/3 -> Mux6/3  "phiIg7"
  Mux6/1 -> Terminator6/1
  Sum2/1 -> Tq/1
  Sum1/1 -> dmEmbScvg/1
  Sum/1 -> dmEmbExh/1
  pMaxFinder/1 -> pMax/1  "pMax"
  pMaxFinder/2 -> Terminator8/1
  EngCylinder_ExtendedOutput/1 -> pCyl/1, pMaxFinder/2  "phiCyl1"
  EngCylinder_ExtendedOutput/9 -> exhVVAOpenCyl/1
  EngCylinder_ExtendedOutput/10 -> vCyl/1
  EngCylinder_ExtendedOutput/11 -> Sum3/1  "dmf1"
  EngCylinder2/9 -> Sum3/2  "dmf2"
  EngCylinder3/9 -> Sum3/3  "dmf3"
  EngCylinder4/9 -> Sum3/4  "dmf4"
  EngCylinder5/9 -> Sum3/5  "dmf5"
  EngCylinder6/9 -> Sum3/6  "dmf6"
  EngCylinder7/9 -> Sum3/7  "dmf7"
  EngCylinder8/9 -> Sum3/8  "dmf8"
  Sum3/1 -> dmf/1  "dmfTot"
  uGov/1 -> Mux8/1
  phiInj/1 -> Mux8/2
  cAStartNom/1 -> Mux8/3
  dCALiftUp/1 -> Mux8/4
  Mux8/1 -> [ctrlSig]
  [ctrlSig] -> Demux/1
  Demux/1 -> EngCylinder_ExtendedOutput/1
  Demux/2 -> EngCylinder_ExtendedOutput/2
  Demux/3 -> EngCylinder_ExtendedOutput/3
  Demux/4 -> EngCylinder_ExtendedOutput/4
  [ctrlSig] -> Demux1/1
  Demux1/1 -> EngCylinder2/1
  Demux1/2 -> EngCylinder2/2
  Demux1/3 -> EngCylinder2/3
  Demux1/4 -> EngCylinder2/4
  [ctrlSig] -> Demux2/1
  Demux2/1 -> EngCylinder3/1
  Demux2/2 -> EngCylinder3/2
  Demux2/3 -> EngCylinder3/3
  Demux2/4 -> EngCylinder3/4
  [ctrlSig] -> Demux3/1
  Demux3/1 -> EngCylinder4/1
  Demux3/2 -> EngCylinder4/2
  Demux3/3 -> EngCylinder4/3
  Demux3/4 -> EngCylinder4/4
  [ctrlSig] -> Demux4/1
  Demux4/1 -> EngCylinder5/1
  Demux4/2 -> EngCylinder5/2
  Demux4/3 -> EngCylinder5/3
  Demux4/4 -> EngCylinder5/4
  [ctrlSig] -> Demux5/1
  Demux5/1 -> EngCylinder6/1
  Demux5/2 -> EngCylinder6/2
  Demux5/3 -> EngCylinder6/3
  Demux5/4 -> EngCylinder6/4
  [ctrlSig] -> Demux6/1
  Demux6/1 -> EngCylinder7/1
  Demux6/2 -> EngCylinder7/2
  Demux6/3 -> EngCylinder7/3
  Demux6/4 -> EngCylinder7/4
  [ctrlSig] -> Demux7/1
  Demux7/1 -> EngCylinder8/1
  Demux7/2 -> EngCylinder8/2
  Demux7/3 -> EngCylinder8/3
  Demux7/4 -> EngCylinder8/4
  EngCylinder2/5 -> Mux1/5  "dmEmbInCyl2"
  EngCylinder3/5 -> Mux2/5  "dmEmbInCyl3"
  EngCylinder4/5 -> Mux3/5  "dmEmbInCyl4"
  EngCylinder5/5 -> Mux4/5  "dmEmbInCyl5"
  EngCylinder6/5 -> Mux5/5  "dmEmbInCyl6"

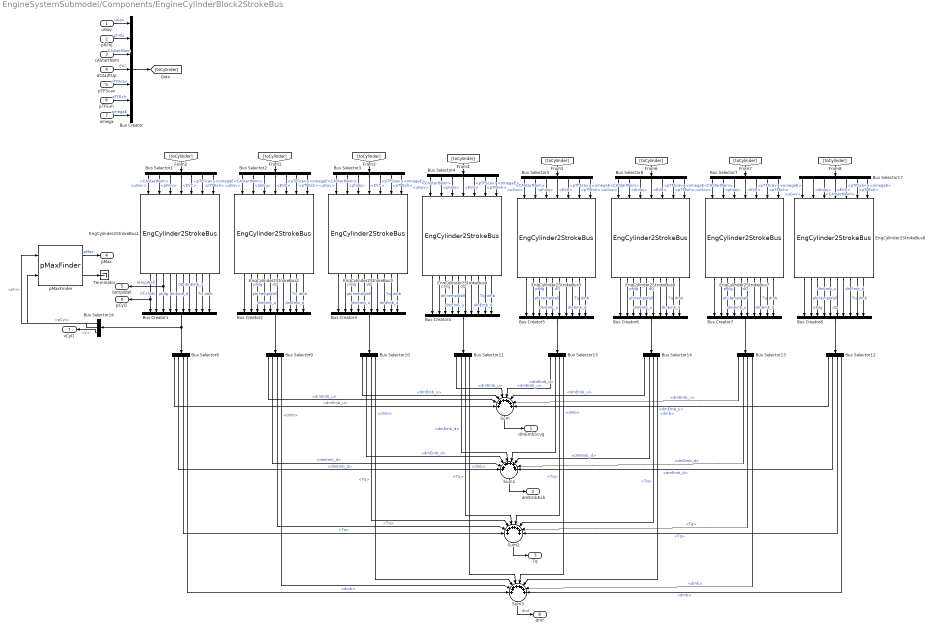
== system EngineSystemSubmodel/Components/EngineCylinderBlock2StrokeBus ==
  uGov : Inport
  phiInj : Inport  Port=2
  cAStartNom : Inport  Port=3
  dCALiftUp : Inport  Port=4
  pTFScav : Inport  Port=5
  pTFExh : Inport  Port=6
  omega : Inport  Port=7
  Bus Creator : BusCreator  Inputs=7
  Bus Creator{1..8} (8 alike) : BusCreator  Inputs=10
  Bus Selector{1..7,17} (8 alike) : BusSelector  OutputSignals=uGov,phiInj,CAStartNom,EVC,pTFScav,pTFExh,omegaE
  Bus Selector{8..15} (8 alike) : BusSelector  OutputSignals=dmEmb_u,dmEmb_d,Tq,dmb
  Bus Selector16 : BusSelector  OutputSignals=pCyl,phi,V
  EngCylinder2StrokeBus1 : EngineSystemSubmodel/Components/EngCylinder2StrokeBus  cylPar=eng.cyl  cylNo=1  cyl=eng.cyl
  EngCylinder2StrokeBus2 : EngineSystemSubmodel/Components/EngCylinder2StrokeBus  cylPar=eng.cyl  cylNo=2  cyl=eng.cyl
  EngCylinder2StrokeBus3 : EngineSystemSubmodel/Components/EngCylinder2StrokeBus  cylPar=eng.cyl  cylNo=3  cyl=eng.cyl
  EngCylinder2StrokeBus4 : EngineSystemSubmodel/Components/EngCylinder2StrokeBus  cylPar=eng.cyl  cylNo=4  cyl=eng.cyl
  EngCylinder2StrokeBus5 : EngineSystemSubmodel/Components/EngCylinder2StrokeBus  cylPar=eng.cyl  cylNo=5  cyl=eng.cyl
  EngCylinder2StrokeBus6 : EngineSystemSubmodel/Components/EngCylinder2StrokeBus  cylPar=eng.cyl  cylNo=6  cyl=eng.cyl
  EngCylinder2StrokeBus7 : EngineSystemSubmodel/Components/EngCylinder2StrokeBus  cylPar=eng.cyl  cylNo=7  cyl=eng.cyl
  EngCylinder2StrokeBus8 : EngineSystemSubmodel/Components/EngCylinder2StrokeBus  cylPar=eng.cyl  cylNo=8  cyl=eng.cyl
  Sum{,1..3} (4 alike) : Sum  Inputs=++++++++
  Terminator : Terminator
  pMaxFinder : EngineSystemSubmodel/EngineOperatingParameterCalculation/pMaxFinder
  dmEmbScvg : Outport
  dmEmbExh : Outport  Port=2
  Tq : Outport  Port=3
  pMax : Outport  Port=4
  tempWall : Outport  Port=5
  pCyl1 : Outport  Port=6
  vCyl1 : Outport  Port=7
  dmf : Outport  Port=8
  wires:
  Bus Selector16/3 -> vCyl1/1  "<V>"
  EngCylinder2StrokeBus1/3 -> tempWall/1, Bus Creator1/3  "tempWall"
  Bus Selector16/2 -> pMaxFinder/1  "<phi>"
  Bus Selector16/1 -> pMaxFinder/2  "<pCyl>"
  Sum3/1 -> dmf/1  "dmf"
  Bus Selector12/4 -> Sum3/8  "<dmb>"
  Bus Selector13/4 -> Sum3/7  "<dmb>"
  Bus Selector14/4 -> Sum3/6  "<dmb>"
  Bus Selector15/4 -> Sum3/5  "<dmb>"
  Bus Selector11/4 -> Sum3/4  "<dmb>"
  Bus Selector10/4 -> Sum3/3  "<dmb>"
  Bus Selector9/4 -> Sum3/2  "<dmb>"
  Bus Selector8/4 -> Sum3/1  "<dmb>"
  Sum2/1 -> Tq/1
  Bus Selector12/3 -> Sum2/8  "<Tq>"
  Bus Selector13/3 -> Sum2/7  "<Tq>"
  Bus Selector14/3 -> Sum2/6  "<Tq>"
  Bus Selector15/3 -> Sum2/5  "<Tq>"
  Bus Selector11/3 -> Sum2/4  "<Tq>"
  Bus Selector10/3 -> Sum2/3  "<Tq>"
  Bus Selector9/3 -> Sum2/2  "<Tq>"
  Bus Selector8/3 -> Sum2/1  "<Tq>"
  Sum1/1 -> dmEmbExh/1
  Bus Selector12/2 -> Sum1/8  "<dmEmb_d>"
  Bus Selector13/2 -> Sum1/7  "<dmEmb_d>"
  Bus Selector14/2 -> Sum1/6  "<dmEmb_d>"
  Bus Selector15/2 -> Sum1/5  "<dmEmb_d>"
  Bus Selector11/2 -> Sum1/4  "<dmEmb_d>"
  Bus Selector10/2 -> Sum1/3  "<dmEmb_d>"
  Bus Selector9/2 -> Sum1/2  "<dmEmb_d>"
  Bus Selector8/2 -> Sum1/1  "<dmEmb_d>"
  Sum/1 -> dmEmbScvg/1
  Bus Selector12/1 -> Sum/8  "<dmEmb_u>"
  Bus Selector13/1 -> Sum/7  "<dmEmb_u>"
  Bus Selector14/1 -> Sum/6  "<dmEmb_u>"
  Bus Selector15/1 -> Sum/5  "<dmEmb_u>"
  Bus Selector11/1 -> Sum/4  "<dmEmb_u>"
  Bus Selector10/1 -> Sum/3  "<dmEmb_u>"
  Bus Selector9/1 -> Sum/2  "<dmEmb_u>"
  Bus Selector8/1 -> Sum/1  "<dmEmb_u>"
  Bus Creator1/1 -> Bus Selector16/1, Bus Selector8/1
  EngCylinder2StrokeBus1/9 -> Bus Creator1/9  "dmb"
  EngCylinder2StrokeBus1/8 -> Bus Creator1/8  "Tq"
  EngCylinder2StrokeBus1/7 -> Bus Creator1/7  "dmEmb_d"
  EngCylinder2StrokeBus1/6 -> Bus Creator1/6  "dmEmb_u"
  EngCylinder2StrokeBus1/5 -> Bus Creator1/5  "dQ"
  EngCylinder2StrokeBus1/4 -> Bus Creator1/4  "phiIg"
  EngCylinder2StrokeBus1/2 -> Bus Creator1/2  "phi"
  EngCylinder2StrokeBus1/1 -> pCyl1/1, Bus Creator1/1  "pCyl"
  Bus Creator/1 -> [toCylinder]
  omega/1 -> Bus Creator/7  "omegaE"
  pTFExh/1 -> Bus Creator/6  "pTFExh"
  pTFScav/1 -> Bus Creator/5  "pTFScav"
  dCALiftUp/1 -> Bus Creator/4  "EVC"
  cAStartNom/1 -> Bus Creator/3  "CAStartNom"
  phiInj/1 -> Bus Creator/2  "phiInj"
  uGov/1 -> Bus Creator/1  "uGov"
  pMaxFinder/2 -> Terminator/1
  pMaxFinder/1 -> pMax/1  "pMax"
  Bus Selector1/6 -> EngCylinder2StrokeBus1/6  "<pTFExh>"
  Bus Selector1/2 -> EngCylinder2StrokeBus1/2  "<phiInj>"
  Bus Selector1/1 -> EngCylinder2StrokeBus1/1  "<uGov>"
  Bus Selector1/4 -> EngCylinder2StrokeBus1/4  "<EVC>"
  Bus Selector1/7 -> EngCylinder2StrokeBus1/7  "<omegaE>"
  Bus Selector1/5 -> EngCylinder2StrokeBus1/5  "<pTFScav>"
  Bus Selector1/3 -> EngCylinder2StrokeBus1/3  "<CAStartNom>"
  [toCylinder] -> Bus Selector1/1
  EngCylinder2StrokeBus1/10 -> Bus Creator1/10
  EngCylinder2StrokeBus2/3 -> Bus Creator2/3  "tempWall"
  Bus Creator2/1 -> Bus Selector9/1
  EngCylinder2StrokeBus2/9 -> Bus Creator2/9  "dmb"
  EngCylinder2StrokeBus2/8 -> Bus Creator2/8  "Tq"
  EngCylinder2StrokeBus2/7 -> Bus Creator2/7  "dmEmb_d"
  EngCylinder2StrokeBus2/6 -> Bus Creator2/6  "dmEmb_u"
  EngCylinder2StrokeBus2/5 -> Bus Creator2/5  "dQ"
  EngCylinder2StrokeBus2/4 -> Bus Creator2/4  "phiIg"
  EngCylinder2StrokeBus2/2 -> Bus Creator2/2  "phi"
  EngCylinder2StrokeBus2/1 -> Bus Creator2/1
  Bus Selector2/6 -> EngCylinder2StrokeBus2/6  "<pTFExh>"
  Bus Selector2/2 -> EngCylinder2StrokeBus2/2  "<phiInj>"
  Bus Selector2/1 -> EngCylinder2StrokeBus2/1  "<uGov>"
  Bus Selector2/4 -> EngCylinder2StrokeBus2/4  "<EVC>"
  Bus Selector2/7 -> EngCylinder2StrokeBus2/7  "<omegaE>"
  Bus Selector2/5 -> EngCylinder2StrokeBus2/5  "<pTFScav>"
  Bus Selector2/3 -> EngCylinder2StrokeBus2/3  "<CAStartNom>"
  [toCylinder] -> Bus Selector2/1
  EngCylinder2StrokeBus2/10 -> Bus Creator2/10
  EngCylinder2StrokeBus3/3 -> Bus Creator3/3  "tempWall"
  Bus Creator3/1 -> Bus Selector10/1
  EngCylinder2StrokeBus3/9 -> Bus Creator3/9  "dmb"
  EngCylinder2StrokeBus3/8 -> Bus Creator3/8  "Tq"
  EngCylinder2StrokeBus3/7 -> Bus Creator3/7  "dmEmb_d"
  EngCylinder2StrokeBus3/6 -> Bus Creator3/6  "dmEmb_u"
  EngCylinder2StrokeBus3/5 -> Bus Creator3/5  "dQ"
  EngCylinder2StrokeBus3/4 -> Bus Creator3/4  "phiIg"
  EngCylinder2StrokeBus3/2 -> Bus Creator3/2  "phi"
  EngCylinder2StrokeBus3/1 -> Bus Creator3/1
  Bus Selector3/6 -> EngCylinder2StrokeBus3/6  "<pTFExh>"
  Bus Selector3/2 -> EngCylinder2StrokeBus3/2  "<phiInj>"
  Bus Selector3/1 -> EngCylinder2StrokeBus3/1  "<uGov>"
  Bus Selector3/4 -> EngCylinder2StrokeBus3/4  "<EVC>"
  Bus Selector3/7 -> EngCylinder2StrokeBus3/7  "<omegaE>"
  Bus Selector3/5 -> EngCylinder2StrokeBus3/5  "<pTFScav>"
  Bus Selector3/3 -> EngCylinder2StrokeBus3/3  "<CAStartNom>"
  [toCylinder] -> Bus Selector3/1
  EngCylinder2StrokeBus3/10 -> Bus Creator3/10
  EngCylinder2StrokeBus4/3 -> Bus Creator4/3  "tempWall"
  Bus Creator4/1 -> Bus Selector11/1
  EngCylinder2StrokeBus4/9 -> Bus Creator4/9  "dmb"
  EngCylinder2StrokeBus4/8 -> Bus Creator4/8  "Tq"
  EngCylinder2StrokeBus4/7 -> Bus Creator4/7  "dmEmb_d"
  EngCylinder2StrokeBus4/6 -> Bus Creator4/6  "dmEmb_u"
  EngCylinder2StrokeBus4/5 -> Bus Creator4/5  "dQ"
  EngCylinder2StrokeBus4/4 -> Bus Creator4/4  "phiIg"
  EngCylinder2StrokeBus4/2 -> Bus Creator4/2  "phi"
  EngCylinder2StrokeBus4/1 -> Bus Creator4/1
  Bus Selector4/6 -> EngCylinder2StrokeBus4/6  "<pTFExh>"
  Bus Selector4/2 -> EngCylinder2StrokeBus4/2  "<phiInj>"
  Bus Selector4/1 -> EngCylinder2StrokeBus4/1  "<uGov>"
  Bus Selector4/4 -> EngCylinder2StrokeBus4/4  "<EVC>"
  Bus Selector4/7 -> EngCylinder2StrokeBus4/7  "<omegaE>"
  Bus Selector4/5 -> EngCylinder2StrokeBus4/5  "<pTFScav>"
  Bus Selector4/3 -> EngCylinder2StrokeBus4/3  "<CAStartNom>"
  [toCylinder] -> Bus Selector4/1
  EngCylinder2StrokeBus4/10 -> Bus Creator4/10
  EngCylinder2StrokeBus5/3 -> Bus Creator5/3  "tempWall"
  Bus Creator5/1 -> Bus Selector15/1
  EngCylinder2StrokeBus5/9 -> Bus Creator5/9  "dmb"
  EngCylinder2StrokeBus5/8 -> Bus Creator5/8  "Tq"
  EngCylinder2StrokeBus5/7 -> Bus Creator5/7  "dmEmb_d"
  EngCylinder2StrokeBus5/6 -> Bus Creator5/6  "dmEmb_u"
  EngCylinder2StrokeBus5/5 -> Bus Creator5/5  "dQ"
  EngCylinder2StrokeBus5/4 -> Bus Creator5/4  "phiIg"
  EngCylinder2StrokeBus5/2 -> Bus Creator5/2  "phi"
  EngCylinder2StrokeBus5/1 -> Bus Creator5/1
  Bus Selector5/6 -> EngCylinder2StrokeBus5/6  "<pTFExh>"
  Bus Selector5/2 -> EngCylinder2StrokeBus5/2  "<phiInj>"
  Bus Selector5/1 -> EngCylinder2StrokeBus5/1  "<uGov>"
  Bus Selector5/4 -> EngCylinder2StrokeBus5/4  "<EVC>"
  Bus Selector5/7 -> EngCylinder2StrokeBus5/7  "<omegaE>"
  Bus Selector5/5 -> EngCylinder2StrokeBus5/5  "<pTFScav>"
  Bus Selector5/3 -> EngCylinder2StrokeBus5/3  "<CAStartNom>"
  [toCylinder] -> Bus Selector5/1
  EngCylinder2StrokeBus5/10 -> Bus Creator5/10
  EngCylinder2StrokeBus6/3 -> Bus Creator6/3  "tempWall"
  Bus Creator6/1 -> Bus Selector14/1
  EngCylinder2StrokeBus6/9 -> Bus Creator6/9  "dmb"
  EngCylinder2StrokeBus6/8 -> Bus Creator6/8  "Tq"
  EngCylinder2StrokeBus6/7 -> Bus Creator6/7  "dmEmb_d"
  EngCylinder2StrokeBus6/6 -> Bus Creator6/6  "dmEmb_u"
  EngCylinder2StrokeBus6/5 -> Bus Creator6/5  "dQ"
  EngCylinder2StrokeBus6/4 -> Bus Creator6/4  "phiIg"
  EngCylinder2StrokeBus6/2 -> Bus Creator6/2  "phi"
  EngCylinder2StrokeBus6/1 -> Bus Creator6/1
  Bus Selector6/6 -> EngCylinder2StrokeBus6/6  "<pTFExh>"
  Bus Selector6/2 -> EngCylinder2StrokeBus6/2  "<phiInj>"
  Bus Selector6/1 -> EngCylinder2StrokeBus6/1  "<uGov>"
  Bus Selector6/4 -> EngCylinder2StrokeBus6/4  "<EVC>"
  Bus Selector6/7 -> EngCylinder2StrokeBus6/7  "<omegaE>"
  Bus Selector6/5 -> EngCylinder2StrokeBus6/5  "<pTFScav>"
  Bus Selector6/3 -> EngCylinder2StrokeBus6/3  "<CAStartNom>"
  [toCylinder] -> Bus Selector6/1
  EngCylinder2StrokeBus6/10 -> Bus Creator6/10
  EngCylinder2StrokeBus7/3 -> Bus Creator7/3  "tempWall"
  Bus Creator7/1 -> Bus Selector13/1
  EngCylinder2StrokeBus7/9 -> Bus Creator7/9  "dmb"
  EngCylinder2StrokeBus7/8 -> Bus Creator7/8  "Tq"
  EngCylinder2StrokeBus7/7 -> Bus Creator7/7  "dmEmb_d"
  EngCylinder2StrokeBus7/6 -> Bus Creator7/6  "dmEmb_u"
  EngCylinder2StrokeBus7/5 -> Bus Creator7/5  "dQ"
  EngCylinder2StrokeBus7/4 -> Bus Creator7/4  "phiIg"
  EngCylinder2StrokeBus7/2 -> Bus Creator7/2  "phi"
  EngCylinder2StrokeBus7/1 -> Bus Creator7/1
  Bus Selector7/6 -> EngCylinder2StrokeBus7/6  "<pTFExh>"
  Bus Selector7/2 -> EngCylinder2StrokeBus7/2  "<phiInj>"
  Bus Selector7/1 -> EngCylinder2StrokeBus7/1  "<uGov>"
  Bus Selector7/4 -> EngCylinder2StrokeBus7/4  "<EVC>"
  Bus Selector7/7 -> EngCylinder2StrokeBus7/7  "<omegaE>"
  Bus Selector7/5 -> EngCylinder2StrokeBus7/5  "<pTFScav>"
  Bus Selector7/3 -> EngCylinder2StrokeBus7/3  "<CAStartNom>"
  [toCylinder] -> Bus Selector7/1
  EngCylinder2StrokeBus7/10 -> Bus Creator7/10
  EngCylinder2StrokeBus8/3 -> Bus Creator8/3  "tempWall"
  Bus Creator8/1 -> Bus Selector12/1
  EngCylinder2StrokeBus8/9 -> Bus Creator8/9  "dmb"
  EngCylinder2StrokeBus8/8 -> Bus Creator8/8  "Tq"
  EngCylinder2StrokeBus8/7 -> Bus Creator8/7  "dmEmb_d"
  EngCylinder2StrokeBus8/6 -> Bus Creator8/6  "dmEmb_u"
  EngCylinder2StrokeBus8/5 -> Bus Creator8/5  "dQ"
  EngCylinder2StrokeBus8/4 -> Bus Creator8/4  "phiIg"
  EngCylinder2StrokeBus8/2 -> Bus Creator8/2  "phi"
  EngCylinder2StrokeBus8/1 -> Bus Creator8/1
  Bus Selector17/6 -> EngCylinder2StrokeBus8/6  "<pTFExh>"
  Bus Selector17/2 -> EngCylinder2StrokeBus8/2  "<phiInj>"
  Bus Selector17/1 -> EngCylinder2StrokeBus8/1  "<uGov>"
  Bus Selector17/4 -> EngCylinder2StrokeBus8/4  "<EVC>"
  Bus Selector17/7 -> EngCylinder2StrokeBus8/7  "<omegaE>"
  Bus Selector17/5 -> EngCylinder2StrokeBus8/5  "<pTFScav>"
  Bus Selector17/3 -> EngCylinder2StrokeBus8/3  "<CAStartNom>"
  [toCylinder] -> Bus Selector17/1
  EngCylinder2StrokeBus8/10 -> Bus Creator8/10

== system EngineSystemSubmodel/Components/EngineCylinderBlock2StrokeBusConv ==
  uGov : Inport
  phiInj : Inport  Port=2
  cAStartNom : Inport  Port=3
  dCALiftUp : Inport  Port=4
  pTFScav : Inport  Port=5
  pTFExh : Inport  Port=6
  omega : Inport  Port=7
  Bus Creator : BusCreator  Inputs=7
  Bus Creator{1..8} (8 alike) : BusCreator  Inputs=10
  Bus Selector{1..7,17} (8 alike) : BusSelector  OutputSignals=uGov,phiInj,CAStartNom,EVC,pTFScav,pTFExh,omegaE
  Bus Selector{8..15} (8 alike) : BusSelector  OutputSignals=dmEmb_u,dmEmb_d,Tq,dmb
  Bus Selector16 : BusSelector  OutputSignals=pCyl,phi,V
  EngCylinder2StrokeBusConv1 : EngineSystemSubmodel/Components/EngCylinder2StrokeBusConv  cylPar=eng.cyl  cylNo=1  cyl=0
  EngCylinder2StrokeBusConv2 : EngineSystemSubmodel/Components/EngCylinder2StrokeBusConv  cylPar=eng.cyl  cylNo=2  cyl=0
  EngCylinder2StrokeBusConv3 : EngineSystemSubmodel/Components/EngCylinder2StrokeBusConv  cylPar=eng.cyl  cylNo=3  cyl=0
  EngCylinder2StrokeBusConv4 : EngineSystemSubmodel/Components/EngCylinder2StrokeBusConv  cylPar=eng.cyl  cylNo=4  cyl=0
  EngCylinder2StrokeBusConv5 : EngineSystemSubmodel/Components/EngCylinder2StrokeBusConv  cylPar=eng.cyl  cylNo=5  cyl=0
  EngCylinder2StrokeBusConv6 : EngineSystemSubmodel/Components/EngCylinder2StrokeBusConv  cylPar=eng.cyl  cylNo=6  cyl=0
  EngCylinder2StrokeBusConv7 : EngineSystemSubmodel/Components/EngCylinder2StrokeBusConv  cylPar=eng.cyl  cylNo=7  cyl=0
  EngCylinder2StrokeBusConv8 : EngineSystemSubmodel/Components/EngCylinder2StrokeBusConv  cylPar=eng.cyl  cylNo=8  cyl=0
  Sum{,1..3} (4 alike) : Sum  Inputs=++++++++
  Terminator : Terminator
  pMaxFinder : EngineSystemSubmodel/EngineOperatingParameterCalculation/pMaxFinder
  dmEmbScvg : Outport
  dmEmbExh : Outport  Port=2
  Tq : Outport  Port=3
  pMax : Outport  Port=4
  tempWall : Outport  Port=5
  pCyl1 : Outport  Port=6
  vCyl1 : Outport  Port=7
  dmf : Outport  Port=8
  wires:
  Bus Selector16/3 -> vCyl1/1  "<V>"
  EngCylinder2StrokeBusConv1/3 -> tempWall/1, Bus Creator1/3  "tempWall"
  Bus Selector16/2 -> pMaxFinder/1  "<phi>"
  Bus Selector16/1 -> pMaxFinder/2  "<pCyl>"
  Sum3/1 -> dmf/1  "dmf"
  Bus Selector12/4 -> Sum3/8  "<dmb>"
  Bus Selector13/4 -> Sum3/7  "<dmb>"
  Bus Selector14/4 -> Sum3/6  "<dmb>"
  Bus Selector15/4 -> Sum3/5  "<dmb>"
  Bus Selector11/4 -> Sum3/4  "<dmb>"
  Bus Selector10/4 -> Sum3/3  "<dmb>"
  Bus Selector9/4 -> Sum3/2  "<dmb>"
  Bus Selector8/4 -> Sum3/1  "<dmb>"
  Sum2/1 -> Tq/1
  Bus Selector12/3 -> Sum2/8  "<Tq>"
  Bus Selector13/3 -> Sum2/7  "<Tq>"
  Bus Selector14/3 -> Sum2/6  "<Tq>"
  Bus Selector15/3 -> Sum2/5  "<Tq>"
  Bus Selector11/3 -> Sum2/4  "<Tq>"
  Bus Selector10/3 -> Sum2/3  "<Tq>"
  Bus Selector9/3 -> Sum2/2  "<Tq>"
  Bus Selector8/3 -> Sum2/1  "<Tq>"
  Sum1/1 -> dmEmbExh/1
  Bus Selector12/2 -> Sum1/8  "<dmEmb_d>"
  Bus Selector13/2 -> Sum1/7  "<dmEmb_d>"
  Bus Selector14/2 -> Sum1/6  "<dmEmb_d>"
  Bus Selector15/2 -> Sum1/5  "<dmEmb_d>"
  Bus Selector11/2 -> Sum1/4  "<dmEmb_d>"
  Bus Selector10/2 -> Sum1/3  "<dmEmb_d>"
  Bus Selector9/2 -> Sum1/2  "<dmEmb_d>"
  Bus Selector8/2 -> Sum1/1  "<dmEmb_d>"
  Sum/1 -> dmEmbScvg/1
  Bus Selector12/1 -> Sum/8  "<dmEmb_u>"
  Bus Selector13/1 -> Sum/7  "<dmEmb_u>"
  Bus Selector14/1 -> Sum/6  "<dmEmb_u>"
  Bus Selector15/1 -> Sum/5  "<dmEmb_u>"
  Bus Selector11/1 -> Sum/4  "<dmEmb_u>"
  Bus Selector10/1 -> Sum/3  "<dmEmb_u>"
  Bus Selector9/1 -> Sum/2  "<dmEmb_u>"
  Bus Selector8/1 -> Sum/1  "<dmEmb_u>"
  Bus Creator1/1 -> Bus Selector16/1, Bus Selector8/1
  EngCylinder2StrokeBusConv1/9 -> Bus Creator1/9  "dmb"
  EngCylinder2StrokeBusConv1/8 -> Bus Creator1/8  "Tq"
  EngCylinder2StrokeBusConv1/7 -> Bus Creator1/7  "dmEmb_d"
  EngCylinder2StrokeBusConv1/6 -> Bus Creator1/6  "dmEmb_u"
  EngCylinder2StrokeBusConv1/5 -> Bus Creator1/5  "dQ"
  EngCylinder2StrokeBusConv1/4 -> Bus Creator1/4  "phiIg"
  EngCylinder2StrokeBusConv1/2 -> Bus Creator1/2  "phi"
  EngCylinder2StrokeBusConv1/1 -> pCyl1/1, Bus Creator1/1  "pCyl"
  Bus Creator/1 -> [toCylinder]
  omega/1 -> Bus Creator/7  "omegaE"
  pTFExh/1 -> Bus Creator/6  "pTFExh"
  pTFScav/1 -> Bus Creator/5  "pTFScav"
  dCALiftUp/1 -> Bus Creator/4  "EVC"
  cAStartNom/1 -> Bus Creator/3  "CAStartNom"
  phiInj/1 -> Bus Creator/2  "phiInj"
  uGov/1 -> Bus Creator/1  "uGov"
  pMaxFinder/2 -> Terminator/1
  pMaxFinder/1 -> pMax/1  "pMax"
  Bus Selector1/6 -> EngCylinder2StrokeBusConv1/6  "<pTFExh>"
  Bus Selector1/2 -> EngCylinder2StrokeBusConv1/2  "<phiInj>"
  Bus Selector1/1 -> EngCylinder2StrokeBusConv1/1  "<uGov>"
  Bus Selector1/4 -> EngCylinder2StrokeBusConv1/4  "<EVC>"
  Bus Selector1/7 -> EngCylinder2StrokeBusConv1/7  "<omegaE>"
  Bus Selector1/5 -> EngCylinder2StrokeBusConv1/5  "<pTFScav>"
  Bus Selector1/3 -> EngCylinder2StrokeBusConv1/3  "<CAStartNom>"
  [toCylinder] -> Bus Selector1/1
  EngCylinder2StrokeBusConv1/10 -> Bus Creator1/10
  EngCylinder2StrokeBusConv2/3 -> Bus Creator2/3  "tempWall"
  Bus Creator2/1 -> Bus Selector9/1
  EngCylinder2StrokeBusConv2/9 -> Bus Creator2/9  "dmb"
  EngCylinder2StrokeBusConv2/8 -> Bus Creator2/8  "Tq"
  EngCylinder2StrokeBusConv2/7 -> Bus Creator2/7  "dmEmb_d"
  EngCylinder2StrokeBusConv2/6 -> Bus Creator2/6  "dmEmb_u"
  EngCylinder2StrokeBusConv2/5 -> Bus Creator2/5  "dQ"
  EngCylinder2StrokeBusConv2/4 -> Bus Creator2/4  "phiIg"
  EngCylinder2StrokeBusConv2/2 -> Bus Creator2/2  "phi"
  EngCylinder2StrokeBusConv2/1 -> Bus Creator2/1
  Bus Selector2/6 -> EngCylinder2StrokeBusConv2/6  "<pTFExh>"
  Bus Selector2/2 -> EngCylinder2StrokeBusConv2/2  "<phiInj>"
  Bus Selector2/1 -> EngCylinder2StrokeBusConv2/1  "<uGov>"
  Bus Selector2/4 -> EngCylinder2StrokeBusConv2/4  "<EVC>"
  Bus Selector2/7 -> EngCylinder2StrokeBusConv2/7  "<omegaE>"
  Bus Selector2/5 -> EngCylinder2StrokeBusConv2/5  "<pTFScav>"
  Bus Selector2/3 -> EngCylinder2StrokeBusConv2/3  "<CAStartNom>"
  [toCylinder] -> Bus Selector2/1
  EngCylinder2StrokeBusConv2/10 -> Bus Creator2/10
  EngCylinder2StrokeBusConv3/3 -> Bus Creator3/3  "tempWall"
  Bus Creator3/1 -> Bus Selector10/1
  EngCylinder2StrokeBusConv3/9 -> Bus Creator3/9  "dmb"
  EngCylinder2StrokeBusConv3/8 -> Bus Creator3/8  "Tq"
  EngCylinder2StrokeBusConv3/7 -> Bus Creator3/7  "dmEmb_d"
  EngCylinder2StrokeBusConv3/6 -> Bus Creator3/6  "dmEmb_u"
  EngCylinder2StrokeBusConv3/5 -> Bus Creator3/5  "dQ"
  EngCylinder2StrokeBusConv3/4 -> Bus Creator3/4  "phiIg"
  EngCylinder2StrokeBusConv3/2 -> Bus Creator3/2  "phi"
  EngCylinder2StrokeBusConv3/1 -> Bus Creator3/1
  Bus Selector3/6 -> EngCylinder2StrokeBusConv3/6  "<pTFExh>"
  Bus Selector3/2 -> EngCylinder2StrokeBusConv3/2  "<phiInj>"
  Bus Selector3/1 -> EngCylinder2StrokeBusConv3/1  "<uGov>"
  Bus Selector3/4 -> EngCylinder2StrokeBusConv3/4  "<EVC>"
  Bus Selector3/7 -> EngCylinder2StrokeBusConv3/7  "<omegaE>"
  Bus Selector3/5 -> EngCylinder2StrokeBusConv3/5  "<pTFScav>"
  Bus Selector3/3 -> EngCylinder2StrokeBusConv3/3  "<CAStartNom>"
  [toCylinder] -> Bus Selector3/1
  EngCylinder2StrokeBusConv3/10 -> Bus Creator3/10
  EngCylinder2StrokeBusConv4/3 -> Bus Creator4/3  "tempWall"
  Bus Creator4/1 -> Bus Selector11/1
  EngCylinder2StrokeBusConv4/9 -> Bus Creator4/9  "dmb"
  EngCylinder2StrokeBusConv4/8 -> Bus Creator4/8  "Tq"
  EngCylinder2StrokeBusConv4/7 -> Bus Creator4/7  "dmEmb_d"
  EngCylinder2StrokeBusConv4/6 -> Bus Creator4/6  "dmEmb_u"
  EngCylinder2StrokeBusConv4/5 -> Bus Creator4/5  "dQ"
  EngCylinder2StrokeBusConv4/4 -> Bus Creator4/4  "phiIg"
  EngCylinder2StrokeBusConv4/2 -> Bus Creator4/2  "phi"
  EngCylinder2StrokeBusConv4/1 -> Bus Creator4/1
  Bus Selector4/6 -> EngCylinder2StrokeBusConv4/6  "<pTFExh>"
  Bus Selector4/2 -> EngCylinder2StrokeBusConv4/2  "<phiInj>"
  Bus Selector4/1 -> EngCylinder2StrokeBusConv4/1  "<uGov>"
  Bus Selector4/4 -> EngCylinder2StrokeBusConv4/4  "<EVC>"
  Bus Selector4/7 -> EngCylinder2StrokeBusConv4/7  "<omegaE>"
  Bus Selector4/5 -> EngCylinder2StrokeBusConv4/5  "<pTFScav>"
  Bus Selector4/3 -> EngCylinder2StrokeBusConv4/3  "<CAStartNom>"
  [toCylinder] -> Bus Selector4/1
  EngCylinder2StrokeBusConv4/10 -> Bus Creator4/10
  EngCylinder2StrokeBusConv5/3 -> Bus Creator5/3  "tempWall"
  Bus Creator5/1 -> Bus Selector15/1
  EngCylinder2StrokeBusConv5/9 -> Bus Creator5/9  "dmb"
  EngCylinder2StrokeBusConv5/8 -> Bus Creator5/8  "Tq"
  EngCylinder2StrokeBusConv5/7 -> Bus Creator5/7  "dmEmb_d"
  EngCylinder2StrokeBusConv5/6 -> Bus Creator5/6  "dmEmb_u"
  EngCylinder2StrokeBusConv5/5 -> Bus Creator5/5  "dQ"
  EngCylinder2StrokeBusConv5/4 -> Bus Creator5/4  "phiIg"
  EngCylinder2StrokeBusConv5/2 -> Bus Creator5/2  "phi"
  EngCylinder2StrokeBusConv5/1 -> Bus Creator5/1
  Bus Selector5/6 -> EngCylinder2StrokeBusConv5/6  "<pTFExh>"
  Bus Selector5/2 -> EngCylinder2StrokeBusConv5/2  "<phiInj>"
  Bus Selector5/1 -> EngCylinder2StrokeBusConv5/1  "<uGov>"
  Bus Selector5/4 -> EngCylinder2StrokeBusConv5/4  "<EVC>"
  Bus Selector5/7 -> EngCylinder2StrokeBusConv5/7  "<omegaE>"
  Bus Selector5/5 -> EngCylinder2StrokeBusConv5/5  "<pTFScav>"
  Bus Selector5/3 -> EngCylinder2StrokeBusConv5/3  "<CAStartNom>"
  [toCylinder] -> Bus Selector5/1
  EngCylinder2StrokeBusConv5/10 -> Bus Creator5/10
  EngCylinder2StrokeBusConv6/3 -> Bus Creator6/3  "tempWall"
  Bus Creator6/1 -> Bus Selector14/1
  EngCylinder2StrokeBusConv6/9 -> Bus Creator6/9  "dmb"
  EngCylinder2StrokeBusConv6/8 -> Bus Creator6/8  "Tq"
  EngCylinder2StrokeBusConv6/7 -> Bus Creator6/7  "dmEmb_d"
  EngCylinder2StrokeBusConv6/6 -> Bus Creator6/6  "dmEmb_u"
  EngCylinder2StrokeBusConv6/5 -> Bus Creator6/5  "dQ"
  EngCylinder2StrokeBusConv6/4 -> Bus Creator6/4  "phiIg"
  EngCylinder2StrokeBusConv6/2 -> Bus Creator6/2  "phi"
  EngCylinder2StrokeBusConv6/1 -> Bus Creator6/1
  Bus Selector6/6 -> EngCylinder2StrokeBusConv6/6  "<pTFExh>"
  Bus Selector6/2 -> EngCylinder2StrokeBusConv6/2  "<phiInj>"
  Bus Selector6/1 -> EngCylinder2StrokeBusConv6/1  "<uGov>"
  Bus Selector6/4 -> EngCylinder2StrokeBusConv6/4  "<EVC>"
  Bus Selector6/7 -> EngCylinder2StrokeBusConv6/7  "<omegaE>"
  Bus Selector6/5 -> EngCylinder2StrokeBusConv6/5  "<pTFScav>"
  Bus Selector6/3 -> EngCylinder2StrokeBusConv6/3  "<CAStartNom>"
  [toCylinder] -> Bus Selector6/1
  EngCylinder2StrokeBusConv6/10 -> Bus Creator6/10
  EngCylinder2StrokeBusConv7/3 -> Bus Creator7/3  "tempWall"
  Bus Creator7/1 -> Bus Selector13/1
  EngCylinder2StrokeBusConv7/9 -> Bus Creator7/9  "dmb"
  EngCylinder2StrokeBusConv7/8 -> Bus Creator7/8  "Tq"
  EngCylinder2StrokeBusConv7/7 -> Bus Creator7/7  "dmEmb_d"
  EngCylinder2StrokeBusConv7/6 -> Bus Creator7/6  "dmEmb_u"
  EngCylinder2StrokeBusConv7/5 -> Bus Creator7/5  "dQ"
  EngCylinder2StrokeBusConv7/4 -> Bus Creator7/4  "phiIg"
  EngCylinder2StrokeBusConv7/2 -> Bus Creator7/2  "phi"
  EngCylinder2StrokeBusConv7/1 -> Bus Creator7/1
  Bus Selector7/6 -> EngCylinder2StrokeBusConv7/6  "<pTFExh>"
  Bus Selector7/2 -> EngCylinder2StrokeBusConv7/2  "<phiInj>"
  Bus Selector7/1 -> EngCylinder2StrokeBusConv7/1  "<uGov>"
  Bus Selector7/4 -> EngCylinder2StrokeBusConv7/4  "<EVC>"
  Bus Selector7/7 -> EngCylinder2StrokeBusConv7/7  "<omegaE>"
  Bus Selector7/5 -> EngCylinder2StrokeBusConv7/5  "<pTFScav>"
  Bus Selector7/3 -> EngCylinder2StrokeBusConv7/3  "<CAStartNom>"
  [toCylinder] -> Bus Selector7/1
  EngCylinder2StrokeBusConv7/10 -> Bus Creator7/10
  EngCylinder2StrokeBusConv8/3 -> Bus Creator8/3  "tempWall"
  Bus Creator8/1 -> Bus Selector12/1
  EngCylinder2StrokeBusConv8/9 -> Bus Creator8/9  "dmb"
  EngCylinder2StrokeBusConv8/8 -> Bus Creator8/8  "Tq"
  EngCylinder2StrokeBusConv8/7 -> Bus Creator8/7  "dmEmb_d"
  EngCylinder2StrokeBusConv8/6 -> Bus Creator8/6  "dmEmb_u"
  EngCylinder2StrokeBusConv8/5 -> Bus Creator8/5  "dQ"
  EngCylinder2StrokeBusConv8/4 -> Bus Creator8/4  "phiIg"
  EngCylinder2StrokeBusConv8/2 -> Bus Creator8/2  "phi"
  EngCylinder2StrokeBusConv8/1 -> Bus Creator8/1
  Bus Selector17/6 -> EngCylinder2StrokeBusConv8/6  "<pTFExh>"
  Bus Selector17/2 -> EngCylinder2StrokeBusConv8/2  "<phiInj>"
  Bus Selector17/1 -> EngCylinder2StrokeBusConv8/1  "<uGov>"
  Bus Selector17/4 -> EngCylinder2StrokeBusConv8/4  "<EVC>"
  Bus Selector17/7 -> EngCylinder2StrokeBusConv8/7  "<omegaE>"
  Bus Selector17/5 -> EngCylinder2StrokeBusConv8/5  "<pTFScav>"
  Bus Selector17/3 -> EngCylinder2StrokeBusConv8/3  "<CAStartNom>"
  [toCylinder] -> Bus Selector17/1
  EngCylinder2StrokeBusConv8/10 -> Bus Creator8/10
